simulink model "Project3"  (R2024b)
settings: Solver=VariableStepAuto  StartTime=0.0  StopTime=100.0  MaxStep=0.01  RelTol=1e-3
undefined symbols (not defined in the file): b, F, k, M
settings Model: Creator=szala  LastModifiedBy=szala

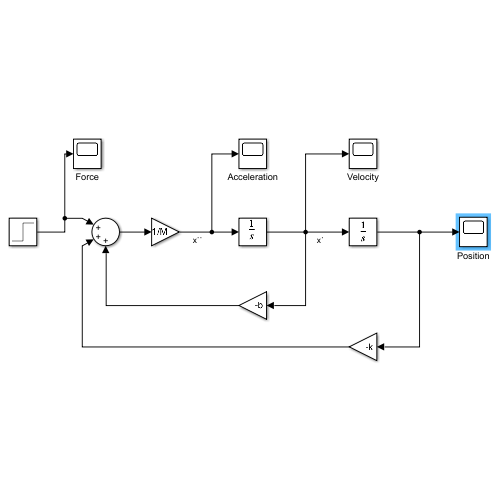
[thumbnail: Simulink's stored preview of the top-level diagram]
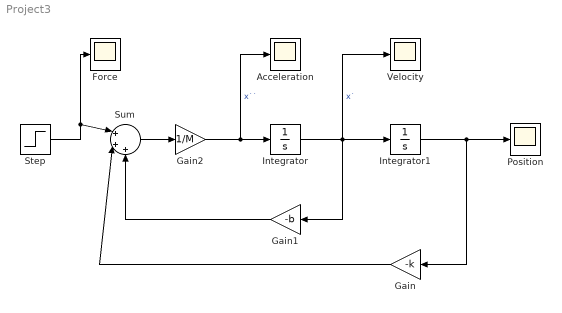
== system Project3 ==
  Acceleration : Scope
  Force : Scope
  Gain : Gain  Gain=-k
  Gain1 : Gain  Gain=-b
  Gain2 : Gain  Gain=1/M
  Integrator : Integrator
  Integrator1 : Integrator
  Position : Scope
  Step : Step  After=F  SampleTime=0
  Sum : Sum  Inputs=|+++
  Velocity : Scope
  wires:
  Integrator/1 -> Gain1/1, Integrator1/1, Velocity/1  "x˙"
  Integrator1/1 -> Gain/1, Position/1
  Step/1 -> Force/1, Sum/1
  Gain1/1 -> Sum/3
  Gain/1 -> Sum/2
  Sum/1 -> Gain2/1
  Gain2/1 -> Acceleration/1, Integrator/1  "x˙˙"
